simulink model "x2tts"  (Simulink 7.3)
settings: Solver=ode45  StartTime=0.0  StopTime=10.0  RelTol=1e-3
libraries: cdsFilt x91, cdsEpicsOut x31, cdsMatrix x4, cdsSwitch x3, cdsWD x3, cdsAdcx0 x1, dac x1, simulink x1, cdsParameters x1
(part 1 of 6)
settings Model: Creator=Jay  LastModifiedBy=jay  ExtModeAutoUpdateStatusClock=off
settings OptimizationCC: InitFltsAndDblsToZero=on

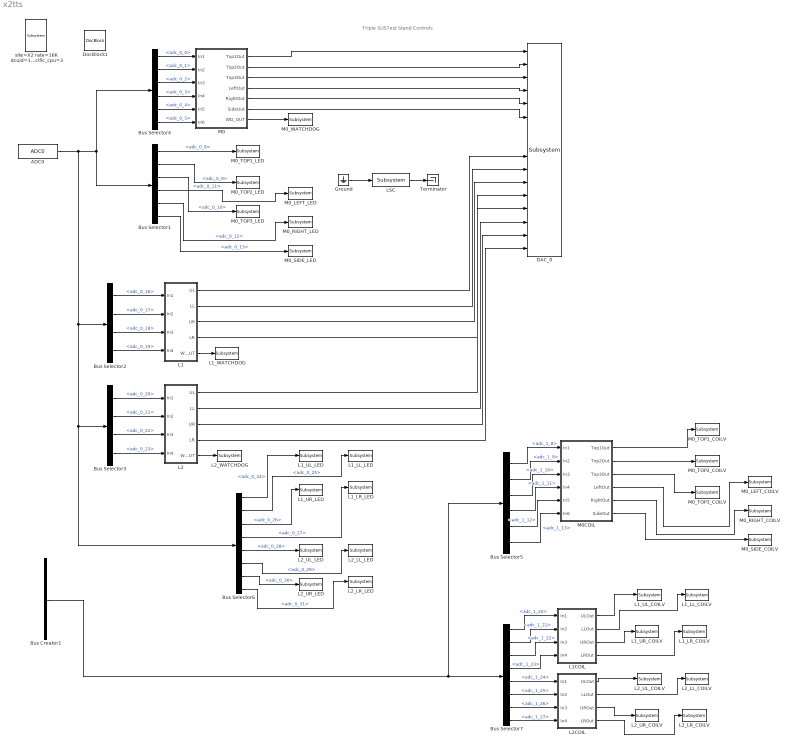
== system x2tts ==
  note: Triple SUSTest Stand Controls
  ADC0 : cdsAdcx0/ADC0  Tag=cdsAdc  Description=|  SystemSampleTime=-1
      | type-GSC_16AI64SSA
      | card_num=0
      settings: AttributesFormatString=%<Description>\n%<Tag>
  Bus Creator1 : BusCreator  Tag=adc_1  Description=|  Inputs='adc_1_0','adc_1_1','adc_1_2','adc_1_3','adc_1_4','adc_1_5','adc_1_6','adc_1_7','adc_1_8','adc_1_9','adc_1_10','adc_1_11','adc_1_12','adc_1_13','adc_1_14','adc_1_15','adc_1_16','adc_1_17','adc_1_18','adc_1_19','adc_1_20','adc_1_21','adc_1_22','adc_1_23','adc_1_24','adc_1_25','adc_1_26','adc_1_27','adc_1_28','adc_1_29','adc_1_30','adc_1_31'
      | PCI66-16AI64SSA
      | 40Vp-p, 16-bit, 610uV/count
      settings: AttributesFormatString=%<Description>\n%<Tag>
  Bus Selector1 : BusSelector  Description=ADC Selector  OutputSignals=adc_0_8,adc_0_9,adc_0_10,adc_0_11,adc_0_12,adc_0_13
      settings: AttributesFormatString=%<Description>
  Bus Selector2 : BusSelector  Description=ADC Selector  OutputSignals=adc_0_16,adc_0_17,adc_0_18,adc_0_19
      settings: AttributesFormatString=%<Description>
  Bus Selector3 : BusSelector  Description=ADC Selector  OutputSignals=adc_0_20,adc_0_21,adc_0_22,adc_0_23
      settings: AttributesFormatString=%<Description>
  Bus Selector4 : BusSelector  Description=ADC Selector  OutputSignals=adc_0_0,adc_0_1,adc_0_2,adc_0_3,adc_0_4,adc_0_5
      settings: AttributesFormatString=%<Description>
  Bus Selector5 : BusSelector  OutputSignals=adc_1_8,adc_1_9,adc_1_10,adc_1_11,adc_1_12,adc_1_13
  Bus Selector6 : BusSelector  OutputSignals=adc_0_24,adc_0_25,adc_0_26,adc_0_27,adc_0_28,adc_0_29,adc_0_30,adc_0_31
  Bus Selector7 : BusSelector  OutputSignals=adc_1_20,adc_1_21,adc_1_22,adc_1_23,adc_1_24,adc_1_25,adc_1_26,adc_1_27
  DAC_0 : dac/Subsystem  Tag=dac_0  Description=|  SystemSampleTime=-1
      | PCI66-16AO16
      | 20Vp-p, 16-bit, 305uV/count
      settings: AttributesFormatString=%<Description>
  DocBlock1 : simulink/Model-Wide Utilities/DocBlock  Tag=SW Install  SystemSampleTime=-1  DocumentType=Text
      settings: AttributesFormatString=%<Tag>
  Ground : Ground
  L1 : Subsystem
  L1COIL : Subsystem
  L1_LL_COILV : cdsEpicsOut/Subsystem  Tag=cdsEpicsOutput  Description=|  SystemSampleTime=-1
      | Purpose:                                          
      | Output a FE signal to an EPICS channel.           
      |                                                   
      | Operation:                                        
      | Takes input value and passes it to EPICS record.  
      |                                                   
      | Usage:                                            
      | Name the part with the desired EPICS rrecord name.
      settings: AttributesFormatString=%<Tag>
  L1_LL_LED : cdsEpicsOut/Subsystem  Tag=cdsEpicsOutput  Description=|  SystemSampleTime=-1
      | Purpose:                                          
      | Output a FE signal to an EPICS channel.           
      |                                                   
      | Operation:                                        
      | Takes input value and passes it to EPICS record.  
      |                                                   
      | Usage:                                            
      | Name the part with the desired EPICS rrecord name.
      settings: AttributesFormatString=%<Tag>
  L1_LR_COILV : cdsEpicsOut/Subsystem  Tag=cdsEpicsOutput  Description=|  SystemSampleTime=-1
      | Purpose:                                          
      | Output a FE signal to an EPICS channel.           
      |                                                   
      | Operation:                                        
      | Takes input value and passes it to EPICS record.  
      |                                                   
      | Usage:                                            
      | Name the part with the desired EPICS rrecord name.
      settings: AttributesFormatString=%<Tag>
  L1_LR_LED : cdsEpicsOut/Subsystem  Tag=cdsEpicsOutput  Description=|  SystemSampleTime=-1
      | Purpose:                                          
      | Output a FE signal to an EPICS channel.           
      |                                                   
      | Operation:                                        
      | Takes input value and passes it to EPICS record.  
      |                                                   
      | Usage:                                            
      | Name the part with the desired EPICS rrecord name.
      settings: AttributesFormatString=%<Tag>
  L1_UL_COILV : cdsEpicsOut/Subsystem  Tag=cdsEpicsOutput  Description=|  SystemSampleTime=-1
      | Purpose:                                          
      | Output a FE signal to an EPICS channel.           
      |                                                   
      | Operation:                                        
      | Takes input value and passes it to EPICS record.  
      |                                                   
      | Usage:                                            
      | Name the part with the desired EPICS rrecord name.
      settings: AttributesFormatString=%<Tag>
  L1_UL_LED : cdsEpicsOut/Subsystem  Tag=cdsEpicsOutput  Description=|  SystemSampleTime=-1
      | Purpose:                                          
      | Output a FE signal to an EPICS channel.           
      |                                                   
      | Operation:                                        
      | Takes input value and passes it to EPICS record.  
      |                                                   
      | Usage:                                            
      | Name the part with the desired EPICS rrecord name.
      settings: AttributesFormatString=%<Tag>
  L1_UR_COILV : cdsEpicsOut/Subsystem  Tag=cdsEpicsOutput  Description=|  SystemSampleTime=-1
      | Purpose:                                          
      | Output a FE signal to an EPICS channel.           
      |                                                   
      | Operation:                                        
      | Takes input value and passes it to EPICS record.  
      |                                                   
      | Usage:                                            
      | Name the part with the desired EPICS rrecord name.
      settings: AttributesFormatString=%<Tag>
  L1_UR_LED : cdsEpicsOut/Subsystem  Tag=cdsEpicsOutput  Description=|  SystemSampleTime=-1
      | Purpose:                                          
      | Output a FE signal to an EPICS channel.           
      |                                                   
      | Operation:                                        
      | Takes input value and passes it to EPICS record.  
      |                                                   
      | Usage:                                            
      | Name the part with the desired EPICS rrecord name.
      settings: AttributesFormatString=%<Tag>
  L1_WATCHDOG : cdsEpicsOut/Subsystem  Tag=cdsEpicsOutput  Description=|  SystemSampleTime=-1
      | Purpose:                                          
      | Output a FE signal to an EPICS channel.           
      |                                                   
      | Operation:                                        
      | Takes input value and passes it to EPICS record.  
      |                                                   
      | Usage:                                            
      | Name the part with the desired EPICS rrecord name.
      settings: AttributesFormatString=%<Tag>
  L2 : Subsystem
  L2COIL : Subsystem
  L2_LL_COILV : cdsEpicsOut/Subsystem  Tag=cdsEpicsOutput  Description=|  SystemSampleTime=-1
      | Purpose:                                          
      | Output a FE signal to an EPICS channel.           
      |                                                   
      | Operation:                                        
      | Takes input value and passes it to EPICS record.  
      |                                                   
      | Usage:                                            
      | Name the part with the desired EPICS rrecord name.
      settings: AttributesFormatString=%<Tag>
  L2_LL_LED : cdsEpicsOut/Subsystem  Tag=cdsEpicsOutput  Description=|  SystemSampleTime=-1
      | Purpose:                                          
      | Output a FE signal to an EPICS channel.           
      |                                                   
      | Operation:                                        
      | Takes input value and passes it to EPICS record.  
      |                                                   
      | Usage:                                            
      | Name the part with the desired EPICS rrecord name.
      settings: AttributesFormatString=%<Tag>
  L2_LR_COILV : cdsEpicsOut/Subsystem  Tag=cdsEpicsOutput  Description=|  SystemSampleTime=-1
      | Purpose:                                          
      | Output a FE signal to an EPICS channel.           
      |                                                   
      | Operation:                                        
      | Takes input value and passes it to EPICS record.  
      |                                                   
      | Usage:                                            
      | Name the part with the desired EPICS rrecord name.
      settings: AttributesFormatString=%<Tag>
  L2_LR_LED : cdsEpicsOut/Subsystem  Tag=cdsEpicsOutput  Description=|  SystemSampleTime=-1
      | Purpose:                                          
      | Output a FE signal to an EPICS channel.           
      |                                                   
      | Operation:                                        
      | Takes input value and passes it to EPICS record.  
      |                                                   
      | Usage:                                            
      | Name the part with the desired EPICS rrecord name.
      settings: AttributesFormatString=%<Tag>
  L2_UL_COILV : cdsEpicsOut/Subsystem  Tag=cdsEpicsOutput  Description=|  SystemSampleTime=-1
      | Purpose:                                          
      | Output a FE signal to an EPICS channel.           
      |                                                   
      | Operation:                                        
      | Takes input value and passes it to EPICS record.  
      |                                                   
      | Usage:                                            
      | Name the part with the desired EPICS rrecord name.
      settings: AttributesFormatString=%<Tag>
  L2_UL_LED : cdsEpicsOut/Subsystem  Tag=cdsEpicsOutput  Description=|  SystemSampleTime=-1
      | Purpose:                                          
      | Output a FE signal to an EPICS channel.           
      |                                                   
      | Operation:                                        
      | Takes input value and passes it to EPICS record.  
      |                                                   
      | Usage:                                            
      | Name the part with the desired EPICS rrecord name.
      settings: AttributesFormatString=%<Tag>
  L2_UR_COILV : cdsEpicsOut/Subsystem  Tag=cdsEpicsOutput  Description=|  SystemSampleTime=-1
      | Purpose:                                          
      | Output a FE signal to an EPICS channel.           
      |                                                   
      | Operation:                                        
      | Takes input value and passes it to EPICS record.  
      |                                                   
      | Usage:                                            
      | Name the part with the desired EPICS rrecord name.
      settings: AttributesFormatString=%<Tag>
  L2_UR_LED : cdsEpicsOut/Subsystem  Tag=cdsEpicsOutput  Description=|  SystemSampleTime=-1
      | Purpose:                                          
      | Output a FE signal to an EPICS channel.           
      |                                                   
      | Operation:                                        
      | Takes input value and passes it to EPICS record.  
      |                                                   
      | Usage:                                            
      | Name the part with the desired EPICS rrecord name.
      settings: AttributesFormatString=%<Tag>
  L2_WATCHDOG : cdsEpicsOut/Subsystem  Tag=cdsEpicsOutput  Description=|  SystemSampleTime=-1
      | Purpose:                                          
      | Output a FE signal to an EPICS channel.           
      |                                                   
      | Operation:                                        
      | Takes input value and passes it to EPICS record.  
      |                                                   
      | Usage:                                            
      | Name the part with the desired EPICS rrecord name.
      settings: AttributesFormatString=%<Tag>
  LSC : cdsFilt/Subsystem  Tag=cdsFilt  Description=|  SystemSampleTime=-1
      | Purpose:                                                                                                                                                                                                                                  
      | Standard CDS IIR filter module.                                                                                                                                                                                                           
      |                                                                                                                                                                                                                                           
      | Operation:                                                                                                                                                                                                                                
      | Consists of 10 second order section IIR filters, plus a ramped gain stage. In FE code, also provides pre-defined test points and excitation channel inputs. The filter coefficients are defined in the LIGO system using the 'foton' tool.
      |                                                                                                                                                                                                                                           
      | Usage:                                                                                                                                                                                                                                    
      | Name the part with the desired filter module name.
      settings: AttributesFormatString=%<Tag>
  M0 : Subsystem
  M0COIL : Subsystem
  M0_LEFT_COILV : cdsEpicsOut/Subsystem  Tag=cdsEpicsOutput  Description=|  SystemSampleTime=-1
      | Purpose:                                          
      | Output a FE signal to an EPICS channel.           
      |                                                   
      | Operation:                                        
      | Takes input value and passes it to EPICS record.  
      |                                                   
      | Usage:                                            
      | Name the part with the desired EPICS rrecord name.
      settings: AttributesFormatString=%<Tag>
  M0_LEFT_LED : cdsEpicsOut/Subsystem  Tag=cdsEpicsOutput  Description=|  SystemSampleTime=-1
      | Purpose:                                          
      | Output a FE signal to an EPICS channel.           
      |                                                   
      | Operation:                                        
      | Takes input value and passes it to EPICS record.  
      |                                                   
      | Usage:                                            
      | Name the part with the desired EPICS rrecord name.
      settings: AttributesFormatString=%<Tag>
  M0_RIGHT_COILV : cdsEpicsOut/Subsystem  Tag=cdsEpicsOutput  Description=|  SystemSampleTime=-1
      | Purpose:                                          
      | Output a FE signal to an EPICS channel.           
      |                                                   
      | Operation:                                        
      | Takes input value and passes it to EPICS record.  
      |                                                   
      | Usage:                                            
      | Name the part with the desired EPICS rrecord name.
      settings: AttributesFormatString=%<Tag>
  M0_RIGHT_LED : cdsEpicsOut/Subsystem  Tag=cdsEpicsOutput  Description=|  SystemSampleTime=-1
      | Purpose:                                          
      | Output a FE signal to an EPICS channel.           
      |                                                   
      | Operation:                                        
      | Takes input value and passes it to EPICS record.  
      |                                                   
      | Usage:                                            
      | Name the part with the desired EPICS rrecord name.
      settings: AttributesFormatString=%<Tag>
  M0_SIDE_COILV : cdsEpicsOut/Subsystem  Tag=cdsEpicsOutput  Description=|  SystemSampleTime=-1
      | Purpose:                                          
      | Output a FE signal to an EPICS channel.           
      |                                                   
      | Operation:                                        
      | Takes input value and passes it to EPICS record.  
      |                                                   
      | Usage:                                            
      | Name the part with the desired EPICS rrecord name.
      settings: AttributesFormatString=%<Tag>
  M0_SIDE_LED : cdsEpicsOut/Subsystem  Tag=cdsEpicsOutput  Description=|  SystemSampleTime=-1
      | Purpose:                                          
      | Output a FE signal to an EPICS channel.           
      |                                                   
      | Operation:                                        
      | Takes input value and passes it to EPICS record.  
      |                                                   
      | Usage:                                            
      | Name the part with the desired EPICS rrecord name.
      settings: AttributesFormatString=%<Tag>
  M0_TOP1_COILV : cdsEpicsOut/Subsystem  Tag=cdsEpicsOutput  Description=|  SystemSampleTime=-1
      | Purpose:                                          
      | Output a FE signal to an EPICS channel.           
      |                                                   
      | Operation:                                        
      | Takes input value and passes it to EPICS record.  
      |                                                   
      | Usage:                                            
      | Name the part with the desired EPICS rrecord name.
      settings: AttributesFormatString=%<Tag>
  M0_TOP1_LED : cdsEpicsOut/Subsystem  Tag=cdsEpicsOutput  Description=|  SystemSampleTime=-1
      | Purpose:                                          
      | Output a FE signal to an EPICS channel.           
      |                                                   
      | Operation:                                        
      | Takes input value and passes it to EPICS record.  
      |                                                   
      | Usage:                                            
      | Name the part with the desired EPICS rrecord name.
      settings: AttributesFormatString=%<Tag>
  M0_TOP2_COILV : cdsEpicsOut/Subsystem  Tag=cdsEpicsOutput  Description=|  SystemSampleTime=-1
      | Purpose:                                          
      | Output a FE signal to an EPICS channel.           
      |                                                   
      | Operation:                                        
      | Takes input value and passes it to EPICS record.  
      |                                                   
      | Usage:                                            
      | Name the part with the desired EPICS rrecord name.
      settings: AttributesFormatString=%<Tag>
  M0_TOP2_LED : cdsEpicsOut/Subsystem  Tag=cdsEpicsOutput  Description=|  SystemSampleTime=-1
      | Purpose:                                          
      | Output a FE signal to an EPICS channel.           
      |                                                   
      | Operation:                                        
      | Takes input value and passes it to EPICS record.  
      |                                                   
      | Usage:                                            
      | Name the part with the desired EPICS rrecord name.
      settings: AttributesFormatString=%<Tag>
  M0_TOP3_COILV : cdsEpicsOut/Subsystem  Tag=cdsEpicsOutput  Description=|  SystemSampleTime=-1
      | Purpose:                                          
      | Output a FE signal to an EPICS channel.           
      |                                                   
      | Operation:                                        
      | Takes input value and passes it to EPICS record.  
      |                                                   
      | Usage:                                            
      | Name the part with the desired EPICS rrecord name.
      settings: AttributesFormatString=%<Tag>
  M0_TOP3_LED : cdsEpicsOut/Subsystem  Tag=cdsEpicsOutput  Description=|  SystemSampleTime=-1
      | Purpose:                                          
      | Output a FE signal to an EPICS channel.           
      |                                                   
      | Operation:                                        
      | Takes input value and passes it to EPICS record.  
      |                                                   
      | Usage:                                            
      | Name the part with the desired EPICS rrecord name.
      settings: AttributesFormatString=%<Tag>
  M0_WATCHDOG : cdsEpicsOut/Subsystem  Tag=cdsEpicsOutput  Description=|  SystemSampleTime=-1
      | Purpose:                                          
      | Output a FE signal to an EPICS channel.           
      |                                                   
      | Operation:                                        
      | Takes input value and passes it to EPICS record.  
      |                                                   
      | Usage:                                            
      | Name the part with the desired EPICS rrecord name.
      settings: AttributesFormatString=%<Tag>
  Terminator : Terminator
  site=X2 rate=16K dcuid=10 host=llosus3 shmem_daq=1 adcSlave=1 specific_cpu=3 : cdsParameters/Subsystem  Tag=cdsParameters  SystemSampleTime=-1
      settings: AttributesFormatString=%<Tag>
  wires:
  Bus Selector4/1 -> M0/1(In1)  "<adc_0_0>"
  Bus Selector4/2 -> M0/2(In2)  "<adc_0_1>"
  Bus Selector4/3 -> M0/3(In3)  "<adc_0_2>"
  Bus Selector4/4 -> M0/4(In4)  "<adc_0_3>"
  Bus Selector4/5 -> M0/5(In5)  "<adc_0_4>"
  Bus Selector4/6 -> M0/6(In6)  "<adc_0_5>"
  ADC0/1 -> Bus Selector4/1, Bus Selector1/1, Bus Selector2/1, Bus Selector3/1, Bus Selector6/1
  M0/1(Top1Out) -> DAC_0/1
  M0/2(Top2Out) -> DAC_0/2
  M0/3(Top3Out) -> DAC_0/3
  M0/4(LeftOut) -> DAC_0/4
  M0/5(RightOut) -> DAC_0/5
  M0/6(SideOut) -> DAC_0/6
  M0/7(WD_OUT) -> M0_WATCHDOG/1
  Bus Selector1/1 -> M0_TOP1_LED/1  "<adc_0_8>"
  Bus Selector1/2 -> M0_TOP2_LED/1  "<adc_0_9>"
  Bus Selector1/3 -> M0_TOP3_LED/1  "<adc_0_10>"
  Bus Selector1/4 -> M0_LEFT_LED/1  "<adc_0_11>"
  Bus Selector1/5 -> M0_RIGHT_LED/1  "<adc_0_12>"
  Bus Selector1/6 -> M0_SIDE_LED/1  "<adc_0_13>"
  M0COIL/1(Top1Out) -> M0_TOP1_COILV/1
  M0COIL/2(Top2Out) -> M0_TOP2_COILV/1
  M0COIL/3(Top3Out) -> M0_TOP3_COILV/1
  M0COIL/4(LeftOut) -> M0_LEFT_COILV/1
  M0COIL/5(RightOut) -> M0_RIGHT_COILV/1
  M0COIL/6(SideOut) -> M0_SIDE_COILV/1
  Bus Creator1/1 -> Bus Selector7/1, Bus Selector5/1
  L1/1(UL) -> DAC_0/9
  L1/2(LL) -> DAC_0/10
  L1/3(UR) -> DAC_0/11
  L1/4(LR) -> DAC_0/12
  L1/5(WD_OUT) -> L1_WATCHDOG/1
  L2/1(UL) -> DAC_0/13
  L2/2(LL) -> DAC_0/14
  L2/3(UR) -> DAC_0/15
  L2/4(LR) -> DAC_0/16
  L2/5(WD_OUT) -> L2_WATCHDOG/1
  Bus Selector6/1 -> L1_UL_LED/1  "<adc_0_24>"
  Bus Selector6/2 -> L1_LL_LED/1  "<adc_0_25>"
  Bus Selector6/3 -> L1_UR_LED/1  "<adc_0_26>"
  Bus Selector6/4 -> L1_LR_LED/1  "<adc_0_27>"
  Bus Selector6/5 -> L2_UL_LED/1  "<adc_0_28>"
  Bus Selector6/6 -> L2_LL_LED/1  "<adc_0_29>"
  Bus Selector6/7 -> L2_UR_LED/1  "<adc_0_30>"
  Bus Selector6/8 -> L2_LR_LED/1  "<adc_0_31>"
  L1COIL/1(ULOut) -> L1_UL_COILV/1
  L1COIL/2(LLOut) -> L1_LL_COILV/1
  L1COIL/3(UROut) -> L1_UR_COILV/1
  L1COIL/4(LROut) -> L1_LR_COILV/1
  L2COIL/1(ULOut) -> L2_UL_COILV/1
  L2COIL/2(LLOut) -> L2_LL_COILV/1
  L2COIL/3(UROut) -> L2_UR_COILV/1
  L2COIL/4(LROut) -> L2_LR_COILV/1
  Ground/1 -> LSC/1
  LSC/1 -> Terminator/1
  Bus Selector2/1 -> L1/1(In1)  "<adc_0_16>"
  Bus Selector2/2 -> L1/2(In2)  "<adc_0_17>"
  Bus Selector2/3 -> L1/3(In3)  "<adc_0_18>"
  Bus Selector2/4 -> L1/4(In4)  "<adc_0_19>"
  Bus Selector3/1 -> L2/1(In1)  "<adc_0_20>"
  Bus Selector3/2 -> L2/2(In2)  "<adc_0_21>"
  Bus Selector3/3 -> L2/3(In3)  "<adc_0_22>"
  Bus Selector3/4 -> L2/4(In4)  "<adc_0_23>"
  Bus Selector7/1 -> L1COIL/1(In1)  "<adc_1_20>"
  Bus Selector7/2 -> L1COIL/2(In2)  "<adc_1_21>"
  Bus Selector7/3 -> L1COIL/3(In3)  "<adc_1_22>"
  Bus Selector7/4 -> L1COIL/4(In4)  "<adc_1_23>"
  Bus Selector7/5 -> L2COIL/1(In1)  "<adc_1_24>"
  Bus Selector7/6 -> L2COIL/2(In2)  "<adc_1_25>"
  Bus Selector7/7 -> L2COIL/3(In3)  "<adc_1_26>"
  Bus Selector7/8 -> L2COIL/4(In4)  "<adc_1_27>"
  Bus Selector5/1 -> M0COIL/1(In1)  "<adc_1_8>"
  Bus Selector5/2 -> M0COIL/2(In2)  "<adc_1_9>"
  Bus Selector5/3 -> M0COIL/3(In3)  "<adc_1_10>"
  Bus Selector5/4 -> M0COIL/4(In4)  "<adc_1_11>"
  Bus Selector5/5 -> M0COIL/5(In5)  "<adc_1_12>"
  Bus Selector5/6 -> M0COIL/6(In6)  "<adc_1_13>"
